simulink model "governor_simulink"  (R2022a)
settings: Solver=ode4  StartTime=0.0  StopTime=t_end  FixedStep=0.1  RelTol=1e-3
values from neighbouring files (symbols this model uses):
  beta = 7    [governor_sim.m]
  dphi0 = 0    [governor_sim.m]
  g = 9.8    [governor_sim.m]
  J = 100    [governor_sim.m]
  k = 10    [governor_sim.m]
  L = 10    [governor_sim.m]
  n = 20    [governor_sim.m]
  omega0 = 0    [governor_sim.m]
  phi0 = pi/4    (= 0.785398163397)    [governor_sim.m]
settings Model: Creator=ntaka  LastModifiedBy=ntaka

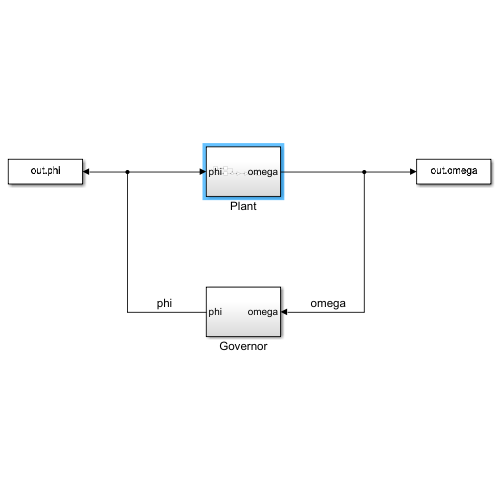
[thumbnail: Simulink's stored preview of the top-level diagram]
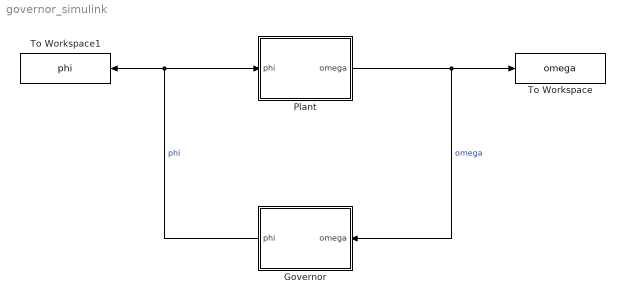
== system governor_simulink ==
  Governor : Subsystem
  Plant : Subsystem
  To Workspace : ToWorkspace  VariableName=omega  SaveFormat=Timeseries  SampleTime=-1
  To Workspace1 : ToWorkspace  VariableName=phi  SaveFormat=Timeseries  SampleTime=-1
  wires:
  Governor/1(phi) -> Plant/1(phi), To Workspace1/1  "phi"
  Plant/1(omega) -> To Workspace/1, Governor/1(omega)  "omega"

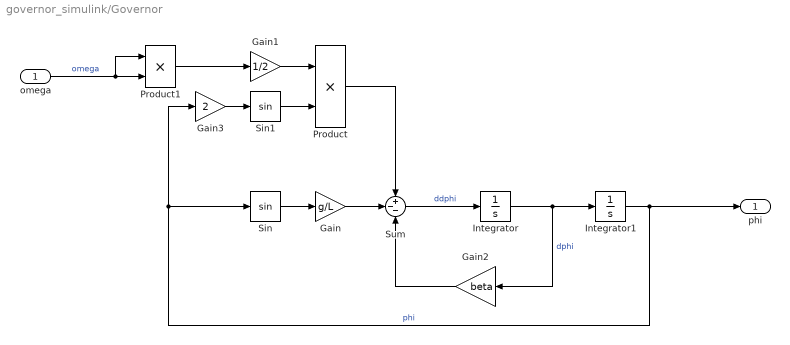
== system governor_simulink/Governor ==
  omega : Inport
  Gain : Gain  Gain=g/L
  Gain1 : Gain  Gain=1/2
  Gain2 : Gain  Gain=beta
  Gain3 : Gain  Gain=2
  Integrator : Integrator  InitialCondition=dphi0
  Integrator1 : Integrator  InitialCondition=phi0
  Product : Product
  Product1 : Product
  Sin : Trigonometry
  Sin1 : Trigonometry
  Sum : Sum  Inputs=+--
  phi : Outport
  wires:
  Integrator1/1 -> Gain3/1, Sin/1, phi/1  "phi"
  Gain/1 -> Sum/2
  Integrator/1 -> Gain2/1, Integrator1/1  "dphi"
  Gain2/1 -> Sum/3
  Sin/1 -> Gain/1
  Sum/1 -> Integrator/1  "ddphi"
  Product1/1 -> Gain1/1
  Gain3/1 -> Sin1/1
  Product/1 -> Sum/1
  omega/1 -> Product1/1, Product1/2  "omega"
  Gain1/1 -> Product/1
  Sin1/1 -> Product/2

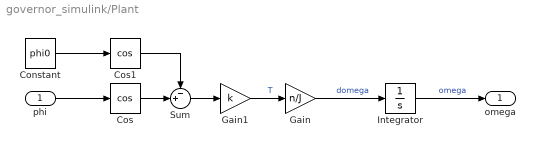
== system governor_simulink/Plant ==
  phi : Inport
  Constant : Constant  Value=phi0
  Cos : Trigonometry  Operator=cos
  Cos1 : Trigonometry  Operator=cos
  Gain : Gain  Gain=n/J
  Gain1 : Gain  Gain=k
  Integrator : Integrator  InitialCondition=omega0
  Sum : Sum  Inputs=-+|
  omega : Outport
  wires:
  Integrator/1 -> omega/1  "omega"
  Cos/1 -> Sum/2
  Gain/1 -> Integrator/1  "domega"
  Gain1/1 -> Gain/1  "T"
  Sum/1 -> Gain1/1
  phi/1 -> Cos/1
  Cos1/1 -> Sum/1
  Constant/1 -> Cos1/1
